simulink model "zad1"  (R2022b)
settings: Solver=FixedStepAuto  StartTime=0.0  StopTime=3  FixedStep=0.00001  RelTol=1e-3
model workspace (MAT data in the model file):
  a0 = 1
  a1 = 1
settings Model: Creator=vandm  LastModifiedBy=vandm

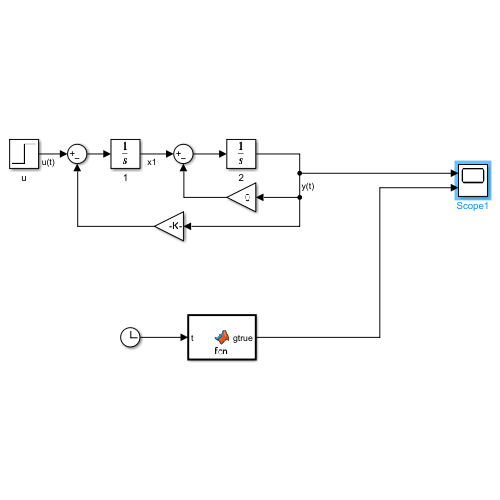
[thumbnail: Simulink's stored preview of the top-level diagram]
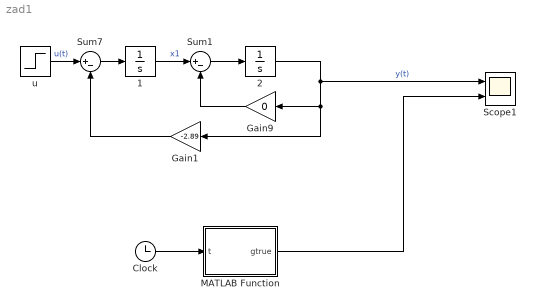
== system zad1 ==
  1 : Integrator  InitialCondition=0.1
  2 : Integrator
  Clock : Clock
  Gain1 : Gain  Gain=-2.89
  Gain9 : Gain  Gain=0
  MATLAB Function : MATLAB Function  TreatAsAtomicUnit=on
  Scope1 : Scope  NumInputPorts=2
  Sum1 : Sum  Inputs=|+-
  Sum7 : Sum  Inputs=|+-
  u : Step  Time=0  After=0  SampleTime=0
  wires:
  u/1 -> Sum7/1  "u(t)"
  Sum7/1 -> 1/1
  1/1 -> Sum1/1  "x1"
  Sum1/1 -> 2/1
  2/1 -> Gain1/1, Gain9/1, Scope1/1  "y(t)"
  Gain9/1 -> Sum1/2
  Gain1/1 -> Sum7/2
  Clock/1 -> MATLAB Function/1(t)
  MATLAB Function/1(gtrue) -> Scope1/2

== matlab function zad1/MATLAB Function ==
  data: t input; gtrue output
function gtrue = fcn(t)

gtrue = (1/34) * exp(1.7 * t) - (1/34) * exp(-1.7 * t);
